simulink model "tetra_mod_qam"  (Simulink 8.0)
settings: Solver=FixedStepDiscrete  SolverMode=SingleTasking  StartTime=0.0  StopTime=1  RelTol=1e-3
undefined symbols (not defined in the file): Fs, get, sided, Two
libraries: commseqgen2 x4, commcnvcod2 x4, commfilt2 x4, commdigbbndam3 x4, commsink2 x4, commchan3 x1, commrandsrc2 x1, commutil2 x1, dspsnks4 x1
settings Model: Creator=tisc1101  LastModifiedBy=Dimav
settings DataIOCC: SignalLoggingSaveFormat=ModelDataLogs
settings DebuggingCC: FcnCallInpInsideContextMsg=UseLocalSettings
settings SFSimCC: SimParseCustomCode=off
settings GRTTargetCC: CombineOutputUpdateFcns=off  GRTInterface=on

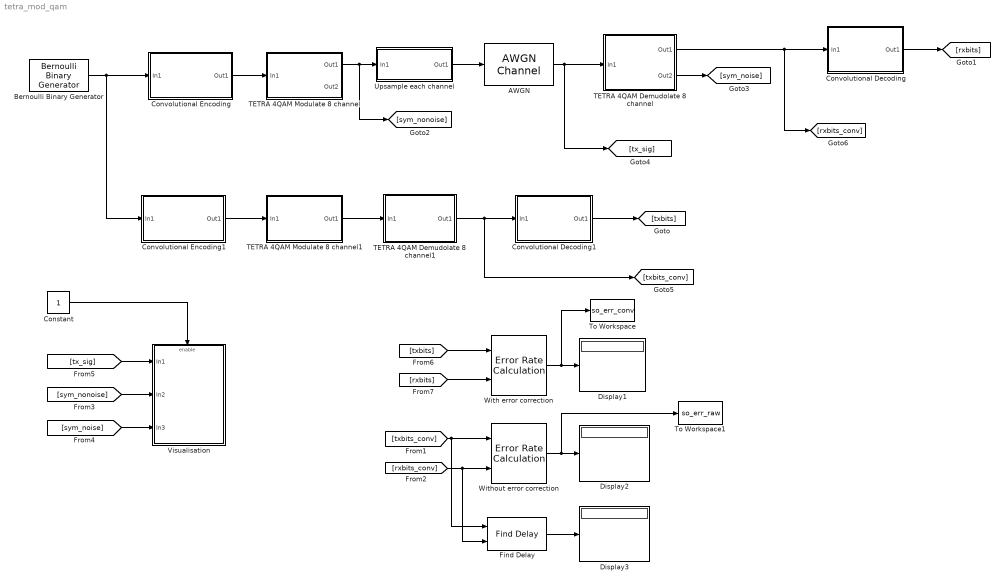
== system tetra_mod_qam ==
  AWGN : commchan3/AWGN Channel  InputProcessing=Columns as channels (frame based)  seed=67  noiseMode="Signal to noise ratio  (SNR)"  EbNodB=10  EsNodB=10  SNRdB=-10  bitsPerSym=1  Ps=1  Tsym=1  variance=1
  Bernoulli Binary Generator : commrandsrc2/Bernoulli Binary Generator  P=0.5  seed=61  Ts=1/(38400/544*200)  frameBased=on  sampPerFrame=200  orient=off  outDataType=double
  Constant : Constant
  Convolutional Decoding : Subsystem
  Convolutional Decoding1 : Subsystem
  Convolutional Encoding : Subsystem
  Convolutional Encoding1 : Subsystem
  Display1 : Display
  Display2 : Display
  Display3 : Display
  Find Delay : commutil2/Find Delay  corrLength=200  chgSigOP=off  stopUpdate=off  numConstDelay=3
  TETRA 4QAM Demudolate 8 channel : Subsystem
  TETRA 4QAM Demudolate 8 channel1 : Subsystem
  TETRA 4QAM Modulate 8 channel : Subsystem
  TETRA 4QAM Modulate 8 channel1 : Subsystem
  To Workspace : ToWorkspace  VariableName=so_err_conv  SampleTime=-1  SaveFormat=Structure
  To Workspace1 : ToWorkspace  VariableName=so_err_raw  SampleTime=-1  SaveFormat=Structure
  Upsample each channel : Subsystem  TreatAsAtomicUnit=on
  Visualisation : Subsystem
  With error correction : commsink2/Error Rate Calculation  N=0  st_delay=0  cp_mode=Entire frame  subframe=[]  PMode=Port  WsName=ErrorVec  RsMode2=off  stop=off  numErr=100  maxBits=1e6
  Without error correction : commsink2/Error Rate Calculation  N=0  st_delay=0  cp_mode=Entire frame  subframe=[]  PMode=Port  WsName=ErrorVec  RsMode2=off  stop=off  numErr=100  maxBits=1e6
  wires:
  [txbits_conv] -> Without error correction/1, Find Delay/1
  [rxbits_conv] -> Without error correction/2, Find Delay/2
  Without error correction/1 -> Display2/1, To Workspace1/1
  TETRA 4QAM Modulate 8 channel/1(Out1) -> Upsample each channel/1(In1), [sym_nonoise]
  TETRA 4QAM Demudolate 8 channel/1(Out1) -> Convolutional Decoding/1(In1), [rxbits_conv]
  TETRA 4QAM Demudolate 8 channel/2(Out2) -> [sym_noise]
  [txbits] -> With error correction/1
  [rxbits] -> With error correction/2
  With error correction/1 -> Display1/1, To Workspace/1
  Bernoulli Binary Generator/1 -> Convolutional Encoding/1(In1), Convolutional Encoding1/1(In1)
  TETRA 4QAM Modulate 8 channel1/1(Out1) -> TETRA 4QAM Demudolate 8 channel1/1(In1)
  TETRA 4QAM Demudolate 8 channel1/1(Out1) -> [txbits_conv], Convolutional Decoding1/1(In1)
  Upsample each channel/1(Out1) -> AWGN/1
  AWGN/1 -> [tx_sig], TETRA 4QAM Demudolate 8 channel/1(In1)
  Convolutional Encoding/1(Out1) -> TETRA 4QAM Modulate 8 channel/1(In1)
  Convolutional Decoding/1(Out1) -> [rxbits]
  Convolutional Encoding1/1(Out1) -> TETRA 4QAM Modulate 8 channel1/1(In1)
  Convolutional Decoding1/1(Out1) -> [txbits]
  Find Delay/1 -> Display3/1
  [tx_sig] -> Visualisation/1(In1)
  [sym_nonoise] -> Visualisation/2(In2)
  [sym_noise] -> Visualisation/3(In3)
  Constant/1 -> Visualisation/Enable

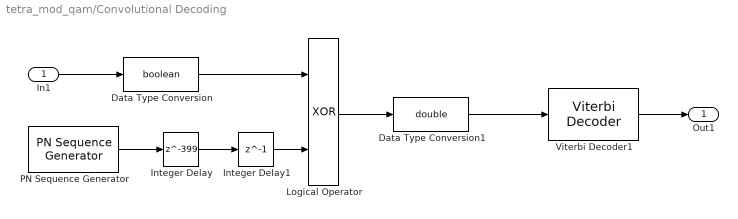
== system tetra_mod_qam/Convolutional Decoding ==
  In1 : Inport
  Data Type Conversion : DataTypeConversion  OutDataTypeStr=boolean
  Data Type Conversion1 : DataTypeConversion  OutDataTypeStr=double
  Integer Delay : Delay  DelayLength=399  InitialCondition=0  InputProcessing=Inherited
  Integer Delay1 : Delay  DelayLength=1  InitialCondition=0  InputProcessing=Inherited
  Logical Operator : Logic  Operator=XOR  AllPortsSameDT=off  OutDataTypeStr=boolean
  PN Sequence Generator : commseqgen2/PN Sequence Generator  poly=[1 1 1 0 1 1 0 1 1 0 1 1 1 0 0 0 1 0 0 0 0 0 1 1 0 0 1 0 0 0 0 0 1]  ini_sta=[0 1 0 1 0 1 0 1 0 1 0 1 0 1 0 1 0 1 0 1 0 1 0 1 0 1 0 1 0 1 1 1]  outBitMaskSource=Dialog parameter  shift=0  outVarSiz=off  maxOutSizeMode=Dialog parameter  maxOutSize=[10 1]  Ts=1/(38400/544*200*2)  frameBased=on  sampPerFrame=400  reset=off  bitPackedOutputs=off  outDataType=boolean  numPackedBits=8  bitPackDataSigned=off  bitPackedOutDType=double
  Viterbi Decoder1 : commcnvcod2/Viterbi Decoder  trellis=poly2trellis(7, [171 133])  isPunctured=off  punctureVector=[1; 1; 0; 1; 0; 1]  erasures=off  dectype=Hard decision  runSigValErrCheck=off  nsdecb=3  smWordLength=16  tbdepth=48  opmode=Continuous  reset=off  outDataType=double  delayedResetAction=off
  Out1 : Outport
  wires:
  Viterbi Decoder1/1 -> Out1/1
  In1/1 -> Data Type Conversion/1
  Data Type Conversion/1 -> Logical Operator/1
  PN Sequence Generator/1 -> Integer Delay/1
  Integer Delay/1 -> Integer Delay1/1
  Integer Delay1/1 -> Logical Operator/2
  Logical Operator/1 -> Data Type Conversion1/1
  Data Type Conversion1/1 -> Viterbi Decoder1/1

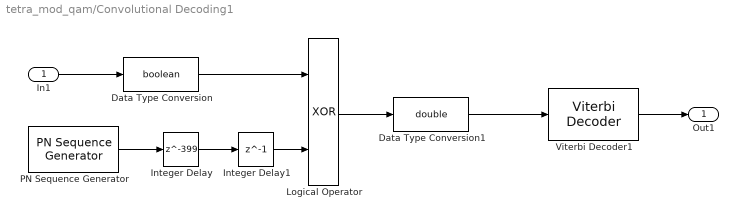
== system tetra_mod_qam/Convolutional Decoding1 ==
  In1 : Inport
  Data Type Conversion : DataTypeConversion  OutDataTypeStr=boolean
  Data Type Conversion1 : DataTypeConversion  OutDataTypeStr=double
  Integer Delay : Delay  DelayLength=399  InitialCondition=0  InputProcessing=Inherited
  Integer Delay1 : Delay  DelayLength=1  InitialCondition=0  InputProcessing=Inherited
  Logical Operator : Logic  Operator=XOR  AllPortsSameDT=off  OutDataTypeStr=boolean
  PN Sequence Generator : commseqgen2/PN Sequence Generator  poly=[1 1 1 0 1 1 0 1 1 0 1 1 1 0 0 0 1 0 0 0 0 0 1 1 0 0 1 0 0 0 0 0 1]  ini_sta=[0 1 0 1 0 1 0 1 0 1 0 1 0 1 0 1 0 1 0 1 0 1 0 1 0 1 0 1 0 1 1 1]  outBitMaskSource=Dialog parameter  shift=0  outVarSiz=off  maxOutSizeMode=Dialog parameter  maxOutSize=[10 1]  Ts=1/(38400/544*200*2)  frameBased=on  sampPerFrame=400  reset=off  bitPackedOutputs=off  outDataType=boolean  numPackedBits=8  bitPackDataSigned=off  bitPackedOutDType=double
  Viterbi Decoder1 : commcnvcod2/Viterbi Decoder  trellis=poly2trellis(7, [171 133])  isPunctured=off  punctureVector=[1; 1; 0; 1; 0; 1]  erasures=off  dectype=Hard decision  runSigValErrCheck=off  nsdecb=3  smWordLength=16  tbdepth=48  opmode=Continuous  reset=off  outDataType=double  delayedResetAction=off
  Out1 : Outport
  wires:
  Viterbi Decoder1/1 -> Out1/1
  In1/1 -> Data Type Conversion/1
  Data Type Conversion/1 -> Logical Operator/1
  PN Sequence Generator/1 -> Integer Delay/1
  Integer Delay/1 -> Integer Delay1/1
  Integer Delay1/1 -> Logical Operator/2
  Logical Operator/1 -> Data Type Conversion1/1
  Data Type Conversion1/1 -> Viterbi Decoder1/1

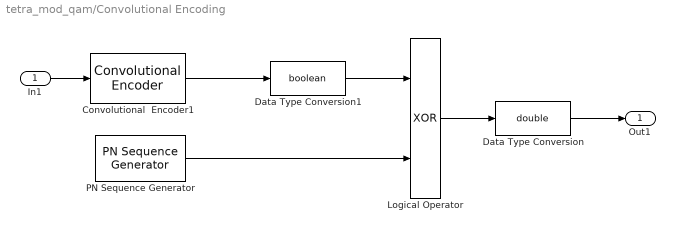
== system tetra_mod_qam/Convolutional Encoding ==
  In1 : Inport
  Convolutional  Encoder1 : commcnvcod2/Convolutional Encoder  trellis=poly2trellis(7, [171 133])  opMode=Continuous  DelayedResetAction=off  hasIniStPort=off  hasFinStPort=off  usePuncVector=off  punctureVector=[1; 1; 0; 1; 0; 1]  reset=Unused parameter value
  Data Type Conversion : DataTypeConversion  OutDataTypeStr=double
  Data Type Conversion1 : DataTypeConversion  OutDataTypeStr=boolean
  Logical Operator : Logic  Operator=XOR  AllPortsSameDT=off  OutDataTypeStr=boolean
  PN Sequence Generator : commseqgen2/PN Sequence Generator  poly=[1 1 1 0 1 1 0 1 1 0 1 1 1 0 0 0 1 0 0 0 0 0 1 1 0 0 1 0 0 0 0 0 1]  ini_sta=[0 1 0 1 0 1 0 1 0 1 0 1 0 1 0 1 0 1 0 1 0 1 0 1 0 1 0 1 0 1 1 1]  outBitMaskSource=Dialog parameter  shift=0  outVarSiz=off  maxOutSizeMode=Dialog parameter  maxOutSize=[10 1]  Ts=1/(38400/544*200*2)  frameBased=on  sampPerFrame=400  reset=off  bitPackedOutputs=off  outDataType=boolean  numPackedBits=8  bitPackDataSigned=off  bitPackedOutDType=double
  Out1 : Outport
  wires:
  In1/1 -> Convolutional  Encoder1/1
  Convolutional  Encoder1/1 -> Data Type Conversion1/1
  Data Type Conversion1/1 -> Logical Operator/1
  Logical Operator/1 -> Data Type Conversion/1
  Data Type Conversion/1 -> Out1/1
  PN Sequence Generator/1 -> Logical Operator/2

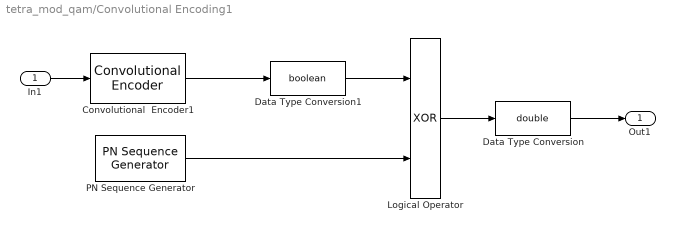
== system tetra_mod_qam/Convolutional Encoding1 ==
  In1 : Inport
  Convolutional  Encoder1 : commcnvcod2/Convolutional Encoder  trellis=poly2trellis(7, [171 133])  opMode=Continuous  DelayedResetAction=off  hasIniStPort=off  hasFinStPort=off  usePuncVector=off  punctureVector=[1; 1; 0; 1; 0; 1]  reset=Unused parameter value
  Data Type Conversion : DataTypeConversion  OutDataTypeStr=double
  Data Type Conversion1 : DataTypeConversion  OutDataTypeStr=boolean
  Logical Operator : Logic  Operator=XOR  AllPortsSameDT=off  OutDataTypeStr=boolean
  PN Sequence Generator : commseqgen2/PN Sequence Generator  poly=[1 1 1 0 1 1 0 1 1 0 1 1 1 0 0 0 1 0 0 0 0 0 1 1 0 0 1 0 0 0 0 0 1]  ini_sta=[0 1 0 1 0 1 0 1 0 1 0 1 0 1 0 1 0 1 0 1 0 1 0 1 0 1 0 1 0 1 1 1]  outBitMaskSource=Dialog parameter  shift=0  outVarSiz=off  maxOutSizeMode=Dialog parameter  maxOutSize=[10 1]  Ts=1/(38400/544*200*2)  frameBased=on  sampPerFrame=400  reset=off  bitPackedOutputs=off  outDataType=boolean  numPackedBits=8  bitPackDataSigned=off  bitPackedOutDType=double
  Out1 : Outport
  wires:
  In1/1 -> Convolutional  Encoder1/1
  Convolutional  Encoder1/1 -> Data Type Conversion1/1
  Data Type Conversion1/1 -> Logical Operator/1
  Logical Operator/1 -> Data Type Conversion/1
  Data Type Conversion/1 -> Out1/1
  PN Sequence Generator/1 -> Logical Operator/2

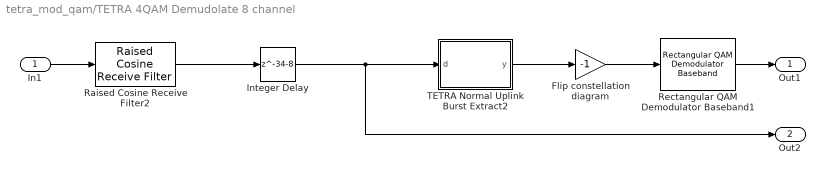
== system tetra_mod_qam/TETRA 4QAM Demudolate 8 channel ==
  In1 : Inport
  Flip constellation diagram : Gain  Gain=-1
  Integer Delay : Delay  DelayLength=34-8  InputProcessing=Columns as channels (frame based)
  Raised Cosine Receive Filter2 : commfilt2/Raised Cosine Receive Filter  filtType=Square root  N=8  D=4  R=0.2  sampMode=Mute  saveAsFlag=0  rateMode=Downsampling  downFactor=8  downOffset=0  framing=Enforce single-rate processing  InputProcessing=Columns as channels (frame based)  checkGain=Normalized  filterGain=1  checkCoeff=off  variableName=rcRxFilt2  launchFVT=off  roundingMode=Floor  overflowMode=off
  Rectangular QAM Demodulator Baseband1 : commdigbbndam3/Rectangular QAM Demodulator Baseband  M=4  PowType=Peak Power  MinDist=2  AvgPow=1  PeakPow=1  Ph=0  Dec=Gray  Mapping=[0:15]  OutType=Bit  DecType=Hard decision  VarSource=Dialog  Variance=1  outDtype1=Inherit via internal rule  outDtype2=Inherit via internal rule  derotateFactorWordLen=16  denormFactorWordLen=16  prodOutWordLen=32  prodOutRoundingMode=Floor  prodOutOverflowMode=Wrap  sumWordLen=32
  TETRA Normal Uplink Burst Extract2 : MATLAB Function  TreatAsAtomicUnit=on
  Out1 : Outport
  Out2 : Outport  Port=2
  wires:
  TETRA Normal Uplink Burst Extract2/1(y) -> Flip constellation diagram/1
  In1/1 -> Raised Cosine Receive Filter2/1
  Rectangular QAM Demodulator Baseband1/1 -> Out1/1
  Flip constellation diagram/1 -> Rectangular QAM Demodulator Baseband1/1
  Raised Cosine Receive Filter2/1 -> Integer Delay/1
  Integer Delay/1 -> TETRA Normal Uplink Burst Extract2/1(d), Out2/1

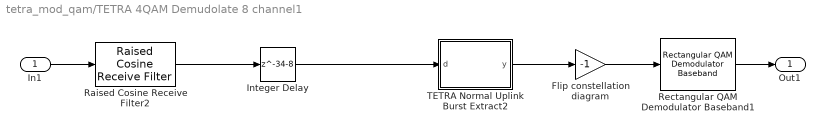
== system tetra_mod_qam/TETRA 4QAM Demudolate 8 channel1 ==
  In1 : Inport
  Flip constellation diagram : Gain  Gain=-1
  Integer Delay : Delay  DelayLength=34-8  InputProcessing=Columns as channels (frame based)
  Raised Cosine Receive Filter2 : commfilt2/Raised Cosine Receive Filter  filtType=Square root  N=8  D=4  R=0.2  sampMode=Mute  saveAsFlag=0  rateMode=Downsampling  downFactor=8  downOffset=0  framing=Enforce single-rate processing  InputProcessing=Columns as channels (frame based)  checkGain=Normalized  filterGain=1  checkCoeff=off  variableName=rcRxFilt2  launchFVT=off  roundingMode=Floor  overflowMode=off
  Rectangular QAM Demodulator Baseband1 : commdigbbndam3/Rectangular QAM Demodulator Baseband  M=4  PowType=Peak Power  MinDist=2  AvgPow=1  PeakPow=1  Ph=0  Dec=Gray  Mapping=[0:15]  OutType=Bit  DecType=Hard decision  VarSource=Dialog  Variance=1  outDtype1=Inherit via internal rule  outDtype2=Inherit via internal rule  derotateFactorWordLen=16  denormFactorWordLen=16  prodOutWordLen=32  prodOutRoundingMode=Floor  prodOutOverflowMode=Wrap  sumWordLen=32
  TETRA Normal Uplink Burst Extract2 : MATLAB Function  TreatAsAtomicUnit=on
  Out1 : Outport
  wires:
  TETRA Normal Uplink Burst Extract2/1(y) -> Flip constellation diagram/1
  In1/1 -> Raised Cosine Receive Filter2/1
  Rectangular QAM Demodulator Baseband1/1 -> Out1/1
  Flip constellation diagram/1 -> Rectangular QAM Demodulator Baseband1/1
  Raised Cosine Receive Filter2/1 -> Integer Delay/1
  Integer Delay/1 -> TETRA Normal Uplink Burst Extract2/1(d)

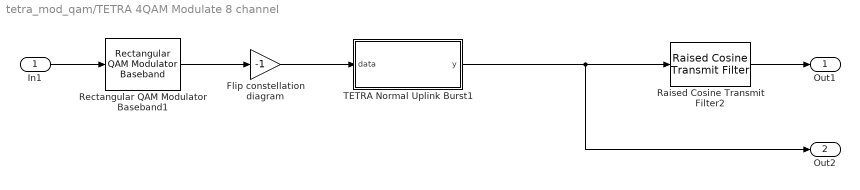
== system tetra_mod_qam/TETRA 4QAM Modulate 8 channel ==
  In1 : Inport
  Flip constellation diagram : Gain  Gain=-1
  Raised Cosine Transmit Filter2 : commfilt2/Raised Cosine Transmit Filter  filtType=Square root  D=4  R=0.2  sampMode=Mute  saveAsFlag=0  N=8  framing=Enforce single-rate processing  InputProcessing=Columns as channels (frame based)  checkGain=Normalized  filterGain=1  checkCoeff=off  variableName=rcTxFilt2  launchFVT=off  roundingMode=Floor  overflowMode=off
  Rectangular QAM Modulator Baseband1 : commdigbbndam3/Rectangular QAM Modulator Baseband  M=4  InType=Bit  Enc=Gray  Mapping=[0:15]  PowType=Peak Power  MinDist=2  AvgPow=1  PeakPow=1  Ph=0  outDtype=double  outWordLen=16  outUDDataType=sfix(16)  outFracLenMode=Best precision  outFracLen=15
  TETRA Normal Uplink Burst1 : MATLAB Function  TreatAsAtomicUnit=on
  Out1 : Outport
  Out2 : Outport  Port=2
  wires:
  Rectangular QAM Modulator Baseband1/1 -> Flip constellation diagram/1
  TETRA Normal Uplink Burst1/1(y) -> Raised Cosine Transmit Filter2/1, Out2/1
  In1/1 -> Rectangular QAM Modulator Baseband1/1
  Raised Cosine Transmit Filter2/1 -> Out1/1
  Flip constellation diagram/1 -> TETRA Normal Uplink Burst1/1(data)

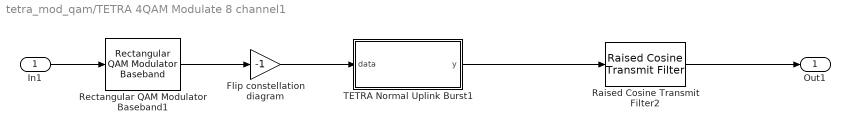
== system tetra_mod_qam/TETRA 4QAM Modulate 8 channel1 ==
  In1 : Inport
  Flip constellation diagram : Gain  Gain=-1
  Raised Cosine Transmit Filter2 : commfilt2/Raised Cosine Transmit Filter  filtType=Square root  D=4  R=0.2  sampMode=Mute  saveAsFlag=0  N=8  framing=Enforce single-rate processing  InputProcessing=Columns as channels (frame based)  checkGain=Normalized  filterGain=1  checkCoeff=off  variableName=rcTxFilt2  launchFVT=off  roundingMode=Floor  overflowMode=off
  Rectangular QAM Modulator Baseband1 : commdigbbndam3/Rectangular QAM Modulator Baseband  M=4  InType=Bit  Enc=Gray  Mapping=[0:15]  PowType=Peak Power  MinDist=2  AvgPow=1  PeakPow=1  Ph=0  outDtype=double  outWordLen=16  outUDDataType=sfix(16)  outFracLenMode=Best precision  outFracLen=15
  TETRA Normal Uplink Burst1 : MATLAB Function  TreatAsAtomicUnit=on
  Out1 : Outport
  wires:
  Rectangular QAM Modulator Baseband1/1 -> Flip constellation diagram/1
  TETRA Normal Uplink Burst1/1(y) -> Raised Cosine Transmit Filter2/1
  In1/1 -> Rectangular QAM Modulator Baseband1/1
  Raised Cosine Transmit Filter2/1 -> Out1/1
  Flip constellation diagram/1 -> TETRA Normal Uplink Burst1/1(data)

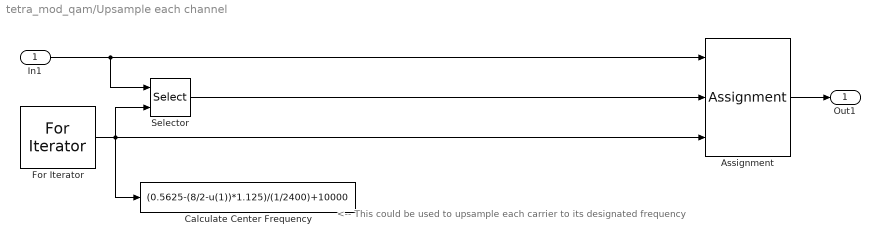
== system tetra_mod_qam/Upsample each channel ==
  note: <--   This could be used to upsample each carrier to its
      | designated frequency
  In1 : Inport
  Assignment : Assignment  NumberOfDimensions=2  IndexMode=Zero-based  IndexOptions=Assign all,Starting index (port)  Indices=1,1  OutputSizes=1,1
  Calculate Center Frequency : Fcn  Expr=(0.5625-(8/2-u(1))*1.125)/(1/2400)+10000
  For Iterator : ForIterator  IterationLimit=8  IndexMode=Zero-based  IterationVariableDataType=double
  Selector : Selector  NumberOfDimensions=2  IndexMode=Zero-based  InputPortWidth=3  IndexOptions=Select all,Starting index (port)  Indices=[1 3],1  OutputSizes=1,1
  Out1 : Outport
  wires:
  In1/1 -> Assignment/1, Selector/1
  For Iterator/1 -> Selector/2, Assignment/3, Calculate Center Frequency/1
  Assignment/1 -> Out1/1
  Selector/1 -> Assignment/2

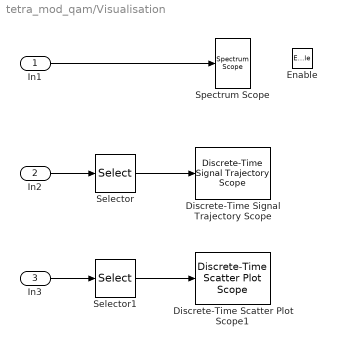
== system tetra_mod_qam/Visualisation ==
  In1 : Inport
  In2 : Inport  Port=2
  In3 : Inport  Port=3
  Enable : EnablePort
  Discrete-Time Scatter Plot Scope1 : commsink2/Discrete-Time Scatter Plot Scope  Tag=ScatterPlot  sampPerSymb=1  offsetEye=0  numTraces=40  numNewFrames=10  LineMarkers=.  LineColors=b  fading=on  render=on  AxisGrid=on  xMin=-1.82571480291123  xMax=2.05872213553488  yMin=-1.92078209044747  yMax=1.96365484799864  inphaseLabel=In-phase Amplitude  quadratureLabel=Quadrature Amplitude  openScopeAtSimStart=on  FrameNumber=off  FigPos=[71 57 560 420]  figTitle=Scatter Plot  numLinesMax=8  block_type_=scatter
  Discrete-Time Signal Trajectory Scope : commsink2/Discrete-Time Signal Trajectory Scope  Tag=SignalTrajectory  sampPerSymb=8  offsetEye=0  numTraces=40  numNewFrames=40  LineStyles=-  LineColors=b  fading=on  render=on  AxisGrid=on  xMin=-0.556680292078565  xMax=0.541832950981133  yMin=-0.549432004547239  yMax=0.54908123851246  inphaseLabel=In-phase Amplitude  quadratureLabel=Quadrature Amplitude  openScopeAtSimStart=on  FrameNumber=off  FigPos=get(0,'defaultfigureposition');  figTitle=Signal Trajectory  numLinesMax=8  block_type_=xy
  Selector : Selector  NumberOfDimensions=2  InputPortWidth=3  IndexOptions=Select all,Starting index (dialog)  Indices=[1 3],1  OutputSizes=1,1
  Selector1 : Selector  NumberOfDimensions=2  InputPortWidth=3  IndexOptions=Select all,Starting index (dialog)  Indices=[1 3],1  OutputSizes=1,1
  Spectrum Scope : dspsnks4/Spectrum Scope  ScopeProperties=on  Domain=Frequency  HorizSpan=1  UseBuffer=off  BufferSize=128  Overlap=64  TreatMby1Signals=One channel  inpFftLenInherit=on  FFTlength=1024  numAvg=5  DisplayProperties=off  AxisGrid=on  Memory=off  FrameNumber=on  AxisLegend=off  AxisZoom=off  OpenScopeAtSimStart=on  OpenScopeImmediately=off  FigPos=[681 44 560 420]  AxisProperties=off  XUnits=Hertz  XRange=Two-sided ((-Fs/2...Fs/2])  XDisplay=0  InheritXIncr=on  XIncr=1.0  XLabel=Samples  XLimit=User-defined  YUnits=dBW/Hertz  XMax=9010.4167  XMin=-8072.9167  YLabel=Magnitude-squared, dB  LineProperties=off  LineDisables=on  LineColors=[0 0 0]  wintypeSpecScope=Hann  RsSpecScope=50  betaSpecScope=5  winsampSpecScope=Periodic  XAxisParamsVer=6.9  isFrameUpgraded=on
      settings: YMin=-105.875  YMax=-33.4583
  wires:
  Selector/1 -> Discrete-Time Signal Trajectory Scope/1
  In3/1 -> Selector1/1
  Selector1/1 -> Discrete-Time Scatter Plot Scope1/1
  In2/1 -> Selector/1
  In1/1 -> Spectrum Scope/1

== matlab function TETRA 4QAM Modulate 8 channel1/TETRA Normal Uplink Burst1 ==
  data: data input double; y output double
function y = qam_frame(data)
%Generate a 4-QAM frame with 8 channels

%Check size
if length(data) < 200
    y=0;
    return;
end

%y=data;
%return;

%Transpose d
d=data';

%Sync symbols from ETSI EN 300 392-2 V3.4.1 (2010-08)
s=zeros(1,16) + 1i * zeros(1,16);
s(1)=exp(1i*0.67190*pi);
s(2)=exp(1i*-0.83201*pi);
s(3)=exp(1i*0.69601*pi);
s(4)=exp(1i*-0.07206*pi);
s(5)=exp(1i*0.07206*pi);
s(6)=exp(1i*-0.69601*pi);
s(7)=exp(1i*0.83201*pi);
s(8)=exp(1i*-0.67190*pi); 
s(9)=exp(1i*0.20310*pi);
s(10)=exp(1i*-0.54299*pi);
s(11)=exp(1i*-0.32101*pi);
s(12)=exp(1i*0.19706*pi);
s(13)=exp(1i*-0.19706*pi);
s(14)=exp(1i*0.32101*pi);
s(15)=exp(1i*0.54299*pi);
s(16)=exp(1i*-0.20310*pi);

%Header symbols are not used
h=zeros(1,8) + 1i + zeros(1,8);

%Pilot symbols from ETSI EN 300 392-2 V3.4.1 (2010-08)
p=zeros(1,24) + 1i * zeros(1,24);
p(1)=exp(1i * -0.90175*pi);
p(2)=exp(1i * 0.38085*pi);
p(3)=exp(1i * 0.64770*pi);
p(4)=exp(1i * 0.97821*pi);
p(5)=exp(1i * 0.97325*pi);
p(6)=exp(1i * -0.24415*pi);
p(7)=exp(1i * 0.27270*pi);
p(8)=exp(1i * 0.10321*pi);
p(9)=exp(1i * -0.15175*pi);
p(10)=exp(1i * 0.13085*pi);
p(11)=exp(1i * 0.89770*pi);
p(12)=exp(1i * 0.22821*pi);
p(13)=exp(1i * -0.77675*pi);
p(14)=exp(1i * -0.99415*pi);
p(15)=exp(1i * 0.02270*pi);
p(16)=exp(1i * 0.85321*pi);
p(17)=exp(1i * -0.40175*pi);
p(18)=exp(1i * 0.88085*pi);
p(19)=exp(1i * 0.14770*pi);
p(20)=exp(1i * 0.47821*pi);
p(21)=exp(1i * 0.09825*pi);
p(22)=exp(1i * -0.61915*pi);
p(23)=exp(1i * -0.35230*pi);
p(24)=exp(1i * -0.02179*pi);

y=[zeros(1,8); zeros(1,8); s(1:8); s(9:16); [d(1) h(1) d(2:5) h(2) d(6)]; d(7:14); d(15:22); d(23:30); [p(1) h(3) p(2) d(31:32) p(3) h(4) p(4)]; d(33:40); d(41:48); d(49:56); d(57:64); [p(5) h(5) p(6) d(65:66) p(7) h(6) p(8)]; d(67:74); d(75:82); d(83:90); d(91:98); [p(9) h(7) p(10) d(99:100) p(11) h(8) p(12)]; d(101:108); d(109:116); d(117:124); d(125:132); [p(13) d(133) p(14) d(134:135) p(15) d(136) p(16)]; d(137:144); d(145:152); d(153:160); d(161:168); [p(17) d(169) p(18) d(170:171) p(19) d(172) p(20)]; d(173:180); d(181:188); d(189:196); [p(21) d(197) p(22) d(198:199) p(23) d(200) p(24)]; zeros(1,8) ];

== matlab function TETRA 4QAM Modulate 8 channel/TETRA Normal Uplink Burst1 ==
  data: data input double; y output double
function y = qam_frame(data)
%Generate a 4-QAM frame with 8 channels

%Check size
if length(data) < 200
    y=0;
    return;
end

%y=data;
%return;

%Transpose d
d=data';

%Sync symbols from ETSI EN 300 392-2 V3.4.1 (2010-08)
s=zeros(1,16) + 1i * zeros(1,16);
s(1)=exp(1i*0.67190*pi);
s(2)=exp(1i*-0.83201*pi);
s(3)=exp(1i*0.69601*pi);
s(4)=exp(1i*-0.07206*pi);
s(5)=exp(1i*0.07206*pi);
s(6)=exp(1i*-0.69601*pi);
s(7)=exp(1i*0.83201*pi);
s(8)=exp(1i*-0.67190*pi); 
s(9)=exp(1i*0.20310*pi);
s(10)=exp(1i*-0.54299*pi);
s(11)=exp(1i*-0.32101*pi);
s(12)=exp(1i*0.19706*pi);
s(13)=exp(1i*-0.19706*pi);
s(14)=exp(1i*0.32101*pi);
s(15)=exp(1i*0.54299*pi);
s(16)=exp(1i*-0.20310*pi);

%Header symbols are not used
h=zeros(1,8) + 1i + zeros(1,8);

%Pilot symbols from ETSI EN 300 392-2 V3.4.1 (2010-08)
p=zeros(1,24) + 1i * zeros(1,24);
p(1)=exp(1i * -0.90175*pi);
p(2)=exp(1i * 0.38085*pi);
p(3)=exp(1i * 0.64770*pi);
p(4)=exp(1i * 0.97821*pi);
p(5)=exp(1i * 0.97325*pi);
p(6)=exp(1i * -0.24415*pi);
p(7)=exp(1i * 0.27270*pi);
p(8)=exp(1i * 0.10321*pi);
p(9)=exp(1i * -0.15175*pi);
p(10)=exp(1i * 0.13085*pi);
p(11)=exp(1i * 0.89770*pi);
p(12)=exp(1i * 0.22821*pi);
p(13)=exp(1i * -0.77675*pi);
p(14)=exp(1i * -0.99415*pi);
p(15)=exp(1i * 0.02270*pi);
p(16)=exp(1i * 0.85321*pi);
p(17)=exp(1i * -0.40175*pi);
p(18)=exp(1i * 0.88085*pi);
p(19)=exp(1i * 0.14770*pi);
p(20)=exp(1i * 0.47821*pi);
p(21)=exp(1i * 0.09825*pi);
p(22)=exp(1i * -0.61915*pi);
p(23)=exp(1i * -0.35230*pi);
p(24)=exp(1i * -0.02179*pi);

y=[zeros(1,8); zeros(1,8); s(1:8); s(9:16); [d(1) h(1) d(2:5) h(2) d(6)]; d(7:14); d(15:22); d(23:30); [p(1) h(3) p(2) d(31:32) p(3) h(4) p(4)]; d(33:40); d(41:48); d(49:56); d(57:64); [p(5) h(5) p(6) d(65:66) p(7) h(6) p(8)]; d(67:74); d(75:82); d(83:90); d(91:98); [p(9) h(7) p(10) d(99:100) p(11) h(8) p(12)]; d(101:108); d(109:116); d(117:124); d(125:132); [p(13) d(133) p(14) d(134:135) p(15) d(136) p(16)]; d(137:144); d(145:152); d(153:160); d(161:168); [p(17) d(169) p(18) d(170:171) p(19) d(172) p(20)]; d(173:180); d(181:188); d(189:196); [p(21) d(197) p(22) d(198:199) p(23) d(200) p(24)]; zeros(1,8) ];

== matlab function TETRA 4QAM Demudolate 8 channel/TETRA Normal Uplink Burst Extract2 ==
  data: d input double; y output double
function y = fcn(d)
%Generate data array from 4QAM-Frame with 8 channels

%Check size
if length(d) < 34
    y=0;
    return;
end

%y=d;
%return;

%Initialize output
temp = zeros(1,200) + 1i * zeros(1,200);

%Extract data from QAM-frame
temp=[d(5,1) d(5,3:6) d(5,8) d(6,1:8) d(7,1:8) d(8,1:8) d(9,4:5) d(10,1:8) d(11,1:8) d(12,1:8) d(13,1:8) d(14,4:5) d(15,1:8) d(16,1:8) d(17,1:8) d(18,1:8) d(19,4:5) d(20,1:8) d(21,1:8) d(22,1:8) d(23,1:8) d(24,2) d(24,4:5) d(24,7) d(25,1:8) d(26,1:8) d(27,1:8) d(28,1:8) d(29,2) d(29,4:5) d(29,7) d(30,1:8) d(31,1:8) d(32,1:8) d(33,2) d(33,4:5) d(33,7) ];
y = temp';

== matlab function TETRA 4QAM Demudolate 8 channel1/TETRA Normal Uplink Burst Extract2 ==
  data: d input double; y output double
function y = fcn(d)
%Generate data array from 4QAM-Frame with 8 channels

%Check size
if length(d) < 34
    y=0;
    return;
end

%y=d;
%return;

%Initialize output
temp = zeros(1,200) + 1i * zeros(1,200);

%Extract data from QAM-frame
temp=[d(5,1) d(5,3:6) d(5,8) d(6,1:8) d(7,1:8) d(8,1:8) d(9,4:5) d(10,1:8) d(11,1:8) d(12,1:8) d(13,1:8) d(14,4:5) d(15,1:8) d(16,1:8) d(17,1:8) d(18,1:8) d(19,4:5) d(20,1:8) d(21,1:8) d(22,1:8) d(23,1:8) d(24,2) d(24,4:5) d(24,7) d(25,1:8) d(26,1:8) d(27,1:8) d(28,1:8) d(29,2) d(29,4:5) d(29,7) d(30,1:8) d(31,1:8) d(32,1:8) d(33,2) d(33,4:5) d(33,7) ];
y = temp';
